simulink model "myAdcSpectrum"  (Simulink 7.3)
settings: Solver=ode45  StartTime=0.0  StopTime=1/fS*5000  RelTol=1e-6
PreLoadFcn:
  | fS = 10000;
  | fN = 75000;
  | fOver = 4;
  | bits = 12;
  | fFilt = 70000;
StopFcn:
  | [analogFreq,analogOut] = myFft0toFs(Analog,fS*2*fOver*5,2,'kHz',0);
  | analogOut = analogOut(1:floor(length(analogOut)/4));
  | analogFreq = analogFreq(1:floor(length(analogFreq)/4));
  | [adcFreq,adcOut] = myFft0toFs(ADC,fS*2*fOver,2,'kHz',0);
  | [dec1Freq,dec1Out] = myFft0toFs(Filt1,fS*2*fOver/2,2,'kHz',0);
  | [dec2Freq,dec2Out] = myFft0toFs(Filt2,fS*2*fOver/4,2,'kHz',0);
  | 
  | scrsz = get(0,'ScreenSize');
  | figure('OuterPosition',[10 scrsz(4)/12 scrsz(3)/1.2 scrsz(4)/1.1])
  | subplot(4,1,1),plot(analogFreq,analogOut)
  | axis([0 fS*fOver*2/1e3 min(analogOut)+5 max(analogOut)+5]);
  | title('Analog Input')
  | subplot(4,1,2),plot(adcFreq,adcOut,'r')
  | axis([0 fS*fOver*2/1e3 min(adcOut)+5 max(adcOut)+5]);
  | title('ADC Output')
  | subplot(4,1,3),plot(dec1Freq,dec1Out,'g')
  | axis([0 fS*fOver*2/1e3 min(dec1Out)+5 max(dec1Out)+5]);
  | title('Decimate Out 1')
  | subplot(4,1,4),plot(dec2Freq,dec2Out,'m')
  | axis([0 fS*fOver*2/1e3 min(dec2Out)+5 max(dec2Out)+5]);
  | title('Decimate Out 2')
libraries: dspmlti4 x2, dsparch4 x1
settings Model: Creator=acarroll  LastModifiedBy=acarroll
settings DataIOCC: LimitDataPoints=off  SaveTime=off
settings DebuggingCC: IntegerOverflowMsg=none

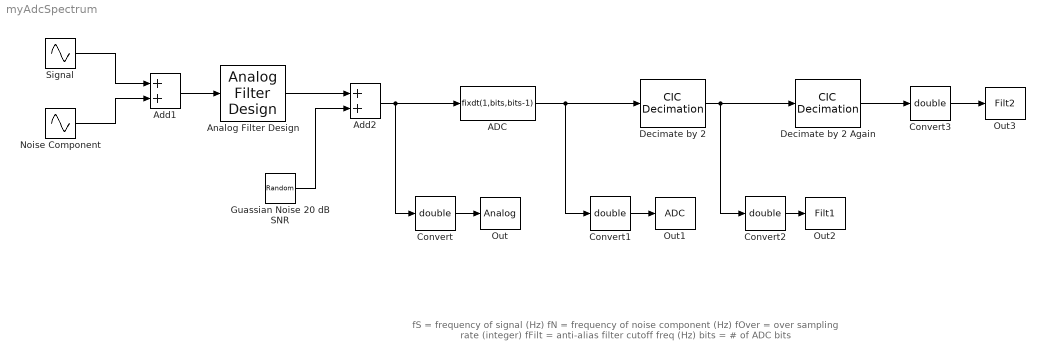
== system myAdcSpectrum ==
  note: fS = frequency of signal (Hz)
      | fN = frequency of noise component (Hz)
      | fOver = over sampling rate (integer)
      | fFilt = anti-alias filter cutoff freq (Hz)
      | bits = # of ADC bits
  ADC : DataTypeConversion  OutDataTypeMode=Specify via dialog  OutDataType=fixdt(1,bits,bits-1)  OutDataTypeStr=fixdt(1,bits,bits-1)  RndMeth=Round  SampleTime=1/fS/fOver/2  SaturateOnIntegerOverflow=on
      settings: AttributesFormatString=Bits = %<OutDataTypeStr>
  Add1 : Sum  OutDataType=fixdt(1, 16)  OutScaling=2^-10
  Add2 : Sum  OutDataType=fixdt(1, 16)  OutScaling=2^-10  SampleTime=1/fS/fOver/2/5
  Analog Filter Design : dsparch4/Analog Filter Design  method=Butterworth  filttype=Lowpass  N=4  Wlo=2*pi*fFilt  Whi=80  Rp=1  Rs=40
  Convert : DataTypeConversion  OutDataTypeMode=double  OutDataType=fixdt(1, 16)  OutScaling=2^0  OutDataTypeStr=double  SampleTime=1/fS/fOver/2/5
  Convert1 : DataTypeConversion  OutDataTypeMode=double  OutDataType=fixdt(1, 16)  OutScaling=2^0  OutDataTypeStr=double  SampleTime=1/fS/fOver/2
  Convert2 : DataTypeConversion  OutDataTypeMode=double  OutDataType=fixdt(1, 16)  OutScaling=2^0  OutDataTypeStr=double
  Convert3 : DataTypeConversion  OutDataTypeMode=double  OutDataType=fixdt(1, 16)  OutScaling=2^0  OutDataTypeStr=double
  Decimate by 2 : dspmlti4/CIC Decimation  DialogController=dspdialog.CICDecimation  filtFrom=Dialog  filtobj=Hm_decim  ftype=Decimator  R=2  M=1  N=4  filterInternals=Full precision  BPS=[16 16 16 16]  FLPS=0  outputWordLength=32  outputFracLength=0  launchFVT=off  framing=Maintain input frame rate
  Decimate by 2 Again : dspmlti4/CIC Decimation  DialogController=dspdialog.CICDecimation  filtFrom=Dialog  filtobj=Hm_decim  ftype=Decimator  R=2  M=1  N=4  filterInternals=Full precision  BPS=[16 16 16 16]  FLPS=0  outputWordLength=32  outputFracLength=0  launchFVT=off  framing=Maintain input frame rate
  Guassian Noise 20 dB SNR : RandomNumber  Variance=(.0354)^2  SampleTime=1/fS/fOver/2/5
  Noise Component : Sin  Amplitude=.5  Bias=0  Frequency=2*pi*fN  Phase=0  Samples=10  SampleTime=0  Offset=0
  Out : ToWorkspace  VariableName=Analog  SampleTime=-1  SaveFormat=Array
  Out1 : ToWorkspace  VariableName=ADC  SampleTime=-1  SaveFormat=Array
  Out2 : ToWorkspace  VariableName=Filt1  SampleTime=-1  SaveFormat=Array
  Out3 : ToWorkspace  VariableName=Filt2  SampleTime=-1  SaveFormat=Array
  Signal : Sin  Amplitude=.5  Bias=0  Frequency=2*pi*fS  Phase=0  Samples=10  SampleTime=0  Offset=0
  wires:
  ADC/1 -> Decimate by 2/1, Convert1/1
  Decimate by 2/1 -> Decimate by 2 Again/1, Convert2/1
  Decimate by 2 Again/1 -> Convert3/1
  Convert2/1 -> Out2/1
  Convert3/1 -> Out3/1
  Signal/1 -> Add1/1
  Noise Component/1 -> Add1/2
  Add1/1 -> Analog Filter Design/1
  Guassian Noise 20 dB SNR/1 -> Add2/2
  Add2/1 -> ADC/1, Convert/1
  Analog Filter Design/1 -> Add2/1
  Convert/1 -> Out/1
  Convert1/1 -> Out1/1
